simulink model "untitled"  (R2015a)
settings: Solver=ode45  StartTime=0.0  StopTime=inf  FixedStep=1  RelTol=1e-3  SampleTimeConstraint=STIndependent
values from neighbouring files (symbols this model uses):
  ee = 0.01    [param.m]
  freq = 50    [param.m]
  Kc = 1.0326    [param.m]
  Kl = 120    [param.m]
  R = 2.4    [param.m]
  Td = 0.324    [param.m]
  Tg = 0.08    [param.m]
  Ti = 1.2116    [param.m]
  Tl = 20    [param.m]
  Tt = 0.3    [param.m]
libraries: simulink x1
settings Model: Creator=BLAGI  LastModifiedBy=BLAGI

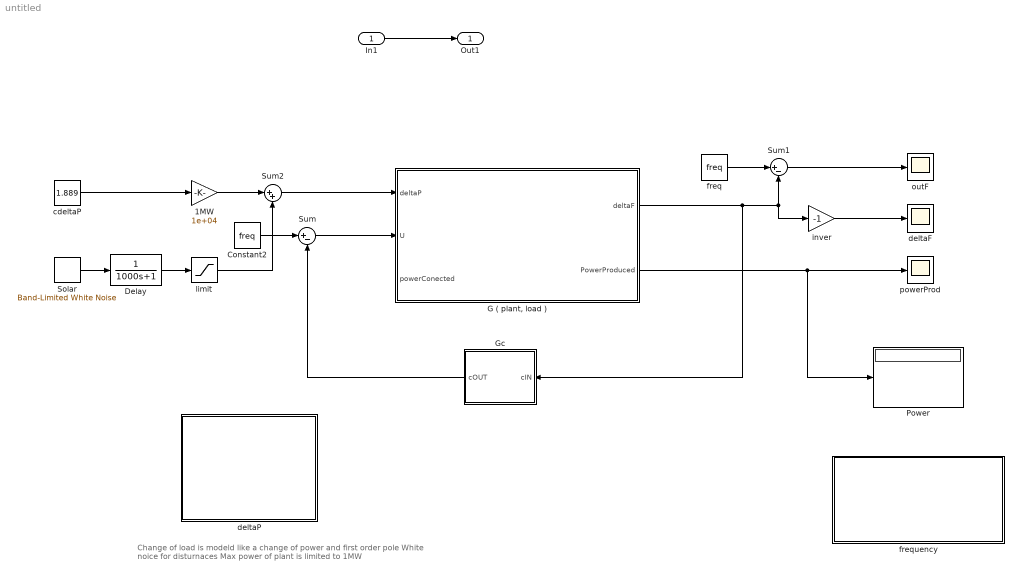
== system untitled ==
  note: Change of load is modeld like a change of power and first order pole
      | White noice for disturnaces
      | Max power of plant is limited to 1MW
  In1 : Inport
  " Solar" : simulink/Sources/Band-Limited White Noise  Cov=[100000]  Ts=0.1  seed=[23341]
  1MW : Gain  Gain=1e+04
  Constant2 : Constant  Value=freq
  Delay : TransferFcn  Denominator=[1000 1]
  "G ( plant, load )" : Subsystem
  "Gc " : Subsystem
  Power : Display
      settings: Format=decimal (Stored Integer)
  Sum : Sum  Inputs=|+-
  Sum1 : Sum  Inputs=|+-
  Sum2 : Sum  Inputs=|++
  cdeltaP : Constant  Value=1.889
  deltaF : Scope
      settings: YMin=-6e-08  YMax=8e-08
  deltaP : Subsystem  DialogController=hmiCreateDDGDialog  IsWebBlock=on  mask(MathWorksWebBlock){webBlockId=c93906c9-f3c1-4ca2-9710-e1dda064d0d9, webBlockType=continuousknob, ShowInLibBrowser=on, ShowInitialText=on, HMISrcModelName=untitled}
      mask prompts: webBlockId "WebBlock Id"; webBlockType "WebBlock Type"; HMISrcModelName "Source Model"
      mask Help: helpview([docroot '/mapfiles/simulink.map'], 'hmi_knob')
      mask Display:
      | if strcmp(get_param(bdroot(gcb),'BlockDiagramType'), 'library')
      |     image([(matlabroot) '/toolbox/simulink/hmi/icons/ContinuousKnob.png']);
      | end
  freq : Constant  Value=freq
  frequency : Subsystem  DialogController=hmiCreateDDGDialog  IsWebBlock=on  mask(MathWorksWebBlock){webBlockId=e5a3aa58-29c8-49de-9c66-e6f9206d89c6, webBlockType=semicirculargauge, ShowInLibBrowser=on, ShowInitialText=on, HMISrcModelName=untitled}
      mask prompts: webBlockId "WebBlock Id"; webBlockType "WebBlock Type"; HMISrcModelName "Source Model"
      mask Help: helpview([docroot '/mapfiles/simulink.map'], 'hmi_half_gauge')
      mask Display:
      | if strcmp(get_param(bdroot(gcb),'BlockDiagramType'), 'library')
      |     image([(matlabroot) '/toolbox/simulink/hmi/icons/SemicircularGauge.png']);
      | end
  inver : Gain  Gain=-1
  limit : Saturate  UpperLimit=1000  LowerLimit=0
  outF : Scope
      settings: YMin=49.6  YMax=50.4
  powerProd : Scope
      settings: YMin=2  YMax=18  SaveName=ScopeData2
  Out1 : Outport
  wires:
  "G ( plant, load )"/1(deltaF) -> "Gc "/1(cIN), inver/1, Sum1/2
  Sum/1 -> "G ( plant, load )"/2(U)
  "Gc "/1(cOUT) -> Sum/2
  Constant2/1 -> Sum/1
  freq/1 -> Sum1/1
  In1/1 -> Out1/1
  inver/1 -> deltaF/1
  cdeltaP/1 -> 1MW/1
  1MW/1 -> Sum2/1
  Sum2/1 -> "G ( plant, load )"/1(deltaP)
  " Solar"/1 -> Delay/1
  Sum1/1 -> outF/1
  "G ( plant, load )"/2(PowerProduced) -> Power/1, powerProd/1
  Delay/1 -> limit/1
  limit/1 -> Sum2/2

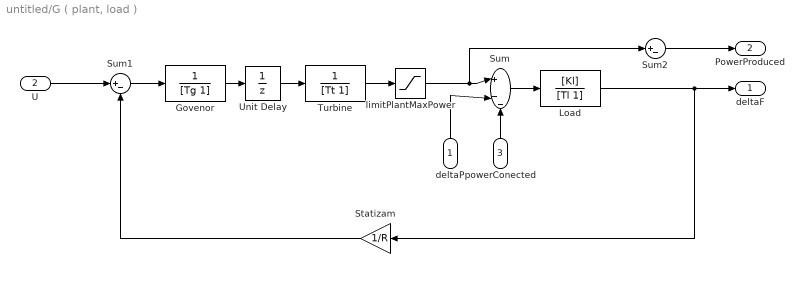
== system untitled/G ( plant, load ) ==
  deltaP : Inport
  U : Inport  Port=2
  powerConected : Inport  Port=3
  Govenor : TransferFcn  Denominator=[Tg 1]
  Load : TransferFcn  Numerator=[Kl]  Denominator=[Tl 1]
  "Statizam " : Gain  Gain=1/R
  Sum : Sum  Inputs=|+--
  Sum1 : Sum  Inputs=|+-
  Sum2 : Sum  Inputs=|+-
  Turbine : TransferFcn  Denominator=[Tt 1]
  Unit Delay : UnitDelay  SampleTime=0.001
  limitPlantMaxPower : Saturate  UpperLimit=1e+7  LowerLimit=0
  deltaF : Outport
  PowerProduced : Outport  Port=2
  wires:
  U/1 -> Sum1/1
  "Statizam "/1 -> Sum1/2
  Govenor/1 -> Unit Delay/1
  Sum/1 -> Load/1
  deltaP/1 -> Sum/2
  Sum1/1 -> Govenor/1
  Turbine/1 -> limitPlantMaxPower/1
  powerConected/1 -> Sum/3
  limitPlantMaxPower/1 -> Sum2/1, Sum/1
  Sum2/1 -> PowerProduced/1
  Unit Delay/1 -> Turbine/1
  Load/1 -> deltaF/1, "Statizam "/1

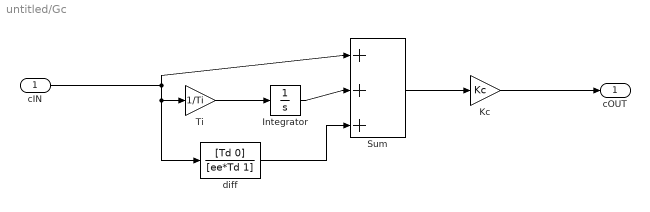
== system untitled/Gc  ==
  cIN : Inport
  Integrator : Integrator
  Kc : Gain  Gain=Kc
  Sum : Sum  Inputs=|+++
  "Ti " : Gain  Gain=1/Ti
  diff : TransferFcn  Numerator=[Td 0]  Denominator=[ee*Td 1]
  cOUT : Outport
  wires:
  cIN/1 -> Sum/1, diff/1, "Ti "/1
  "Ti "/1 -> Integrator/1
  Sum/1 -> Kc/1
  diff/1 -> Sum/3
  Integrator/1 -> Sum/2
  Kc/1 -> cOUT/1

== system untitled/deltaP ==

== system untitled/frequency ==
